simulink model "puntoc"  (R2020a)
settings: Solver=VariableStepAuto  StartTime=0.0  StopTime=10.0  RelTol=1e-3
settings Model: Creator=Usuario  LastModifiedBy=Usuario

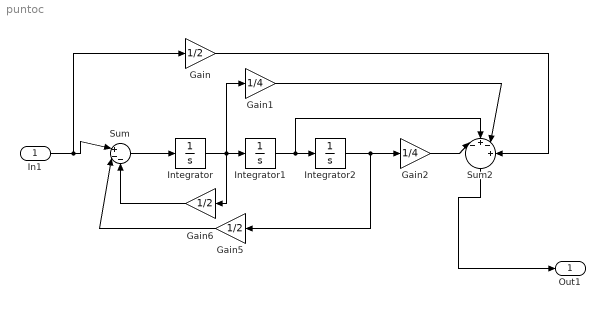
== system puntoc ==
  In1 : Inport
  Gain : Gain  Gain=1/2
  Gain1 : Gain  Gain=1/4
  Gain2 : Gain  Gain=1/4
  Gain5 : Gain  Gain=1/2
  Gain6 : Gain  Gain=1/2
  Integrator : Integrator
  Integrator1 : Integrator
  Integrator2 : Integrator
  Sum : Sum  Inputs=|+--
  Sum2 : Sum  Inputs=|-+-+
  Out1 : Outport
  wires:
  In1/1 -> Gain/1, Sum/1
  Integrator/1 -> Gain1/1, Gain6/1, Integrator1/1
  Integrator1/1 -> Sum2/2, Integrator2/1
  Sum/1 -> Integrator/1
  Sum2/1 -> Out1/1
  Gain/1 -> Sum2/4
  Gain1/1 -> Sum2/3
  Integrator2/1 -> Gain5/1, Gain2/1
  Gain2/1 -> Sum2/1
  Gain5/1 -> Sum/2
  Gain6/1 -> Sum/3
